simulink model "UAV_Research_Environment"  (R2025a)
settings: Solver=ode23t  StartTime=0.0  StopTime=130  MaxStep=2e-3  RelTol=1e-4  AbsTol=1e-3  EnableMultiTasking=on
InitFcn:
  | skipInitialization = false;
  | 
  | if evalin('base', ...
  |         'exist(''CONTROLLER_TUNING_ACTIVE'',''var'')')
  | 
  |     skipInitialization = evalin('base', ...
  |         'logical(CONTROLLER_TUNING_ACTIVE)');
  | end
  | 
  | if ~skipInitialization
  | 
  |     icraControllerPrepared = false;
  | 
  |     hasICRAVariables = evalin('base', ...
  |         ['exist(''AUTOPILOT'',''var'') && ' ...
  |          'exist(''ICRA_ACTIVE_CONTROLLER'',''var'') && ' ...
  |          'exist(''ICRA_ACTIVE_RUN_ID'',''var'')']);
  | 
  |     if hasICRAVariables
  | 
  |         icraControllerPrepared = evalin('base', ...
  |             ['isstruct(AUTOPILOT) && ' ...
  |              'isfield(AUTOPILOT,''info'') && ' ...
  |              'isfield(AUTOPILOT.info,''ICRAControllerID'') && ' ...
  |              'strcmp(string(AUTOPILOT.info.ICRAControllerID), ' ...
  |                     'string(ICRA_ACTIVE_CONTROLLER))']);
  | 
  |     end
  | 
  |     if icraControllerPrepared
  |         skipInitialization = true;
  |     end
  | end
  | 
  | if ~skipInitialization
  | 
  |     mdl = bdroot;
  | 
  |     mdl_file = get_param(mdl, 'FileName');
  | 
  |     project_root = fileparts(mdl_file);
  | 
  |     init_file = fullfile(project_root, 'initialize_project.m');
  | 
  |     if exist(init_file, 'file')
  | 
  |         run(init_file);
  | 
  |     else
  | 
  |         error('initialize_project.m was not found in the model folder.');
  | 
  |     end
  | end
values from neighbouring files (symbols this model uses):
  A_UAV = struct()    [UAV_analytical.m]
  AUTOPILOT = struct()    [UAV_autopilot.m]
  B_UAV = struct()    [UAV_block.m]
  D = A_UAV.source.propeller_diameter_m    [UAV_analytical.m]    (also in plot_controller_results.m = permute(                  D,                  order); plot_estimator_results.m = permute(              D,              order); plot_mission_results.m = permute(                  D,                  order); plot_touchdown_diagnostics.m = permute(                  D,                  order))
  OPERATOR_MODE = OPERATOR_MODE_MANUAL    [initialize_project.m]    (also in uav_remote_gui.m = uint8(0))
  P_ENV = struct()    [Environment.m]
  P_UAV = struct()    [UAV_simscape.m]
  s = sin(angle)    [uav_remote_gui.m]
  SENSOR = struct()    [UAV_sensors.m]
  TRAJECTORY_CONFIG = struct()    [UAV_trajectories.m]
  TRAJECTORY_ID = uint8(          trajectoryIDNumeric)    [UAV_trajectories.m]
  X = reshape(                  D,                  nt,                  [])    [plot_controller_results.m]    (also in plot_estimator_results.m = reshape(              D,              nt,              []); plot_mission_results.m; plot_touchdown_diagnostics.m; plot_trajectory_3d.m)
  Y = absolutePlanNED(1,:)    [plot_trajectory_3d.m]    (also in uav_remote_gui.m = positionNED(:,1))
  Z = landedCGDown -          absolutePlanNED(3,:)    [plot_trajectory_3d.m]    (also in uav_remote_gui.m = landedCGDown-positionNED(:,3))
undefined symbols (not defined in the file or in its folder): Acceleration_ref, F, fractalcoef, Light, MIL, Position_ref, Velocity_ref, Yaw_ref, YawRate_ref
libraries: sm_lib x49, nesl_utility x29, fl_lib x17, slpidlib x16, simulink x14, ee_lib x5, sdl_lib x4, aerolibwind2 x3, aerolibatmos2 x2, sensorbarometerlib x1, sensorgpslib x1, mspsensorlib x1
(part 9 of 9)

== matlab function UAV_Research_Environment/State Estimator/Navigation_Health ==
  data: HealthFlags input; NavValid output; StateStd input; InnovationSigma input; NavHealthStatus output; ESTIMATOR parameter
function [NavValid, NavHealthStatus] = ...
    Navigation_Health(HealthFlags, StateStd, InnovationSigma, ESTIMATOR)
persistent gpsSamplesSinceUpdate
persistent magSamplesSinceUpdate
persistent baroSamplesSinceUpdate
persistent gpsUpdateObserved
persistent magUpdateObserved
persistent baroUpdateObserved
persistent gpsInnovationHealthyLatched
persistent magInnovationHealthyLatched
persistent baroInnovationHealthyLatched
persistent healthyCounter
persistent unhealthyCounter
persistent navValidLatched
Ts = ...
    ESTIMATOR.rate.imuSampleTime_s;
gpsTimeoutSamples = ...
    uint32(ceil( ...
        ESTIMATOR.health.gpsTimeout_s / Ts));
magTimeoutSamples = ...
    uint32(ceil( ...
        ESTIMATOR.health.magTimeout_s / Ts));
baroTimeoutSamples = ...
    uint32(ceil( ...
        ESTIMATOR.health.baroTimeout_s / Ts));
validConfirmationSamples = ...
    uint32(ceil( ...
        ESTIMATOR.health.validConfirmationTime_s / Ts));
invalidConfirmationSamples = ...
    uint32(ceil( ...
        ESTIMATOR.health.invalidConfirmationTime_s / Ts));
if isempty(navValidLatched)
    gpsSamplesSinceUpdate = ...
        gpsTimeoutSamples + uint32(1);
    magSamplesSinceUpdate = ...
        magTimeoutSamples + uint32(1);
    baroSamplesSinceUpdate = ...
        baroTimeoutSamples + uint32(1);
    gpsUpdateObserved = ...
        false;
    magUpdateObserved = ...
        false;
    baroUpdateObserved = ...
        false;
    gpsInnovationHealthyLatched = ...
        false;
    magInnovationHealthyLatched = ...
        false;
    baroInnovationHealthyLatched = ...
        false;
    healthyCounter = ...
        uint32(0);
    unhealthyCounter = ...
        uint32(0);
    navValidLatched = ...
        false;
end
EstimatorInitialized = ...
    logical(HealthFlags(1));
IMUInputValid = ...
    logical(HealthFlags(2));
GPSInputValid = ...
    logical(HealthFlags(3));
MagInputValid = ...
    logical(HealthFlags(4));
BaroInputValid = ...
    logical(HealthFlags(5));
GPSUpdate = ...
    logical(HealthFlags(6));
MagUpdate = ...
    logical(HealthFlags(7));
BaroUpdate = ...
    logical(HealthFlags(8));
StateFinite = ...
    logical(HealthFlags(9));
CovarianceFinite = ...
    logical(HealthFlags(10));
QuaternionValid = ...
    logical(HealthFlags(11));
if ~EstimatorInitialized
    gpsSamplesSinceUpdate = ...
        gpsTimeoutSamples + uint32(1);
    magSamplesSinceUpdate = ...
        magTimeoutSamples + uint32(1);
    baroSamplesSinceUpdate = ...
        baroTimeoutSamples + uint32(1);
    gpsUpdateObserved = ...
        false;
    magUpdateObserved = ...
        false;
    baroUpdateObserved = ...
        false;
    gpsInnovationHealthyLatched = ...
        false;
    magInnovationHealthyLatched = ...
        false;
    baroInnovationHealthyLatched = ...
        false;
    healthyCounter = ...
        uint32(0);
    unhealthyCounter = ...
        uint32(0);
    navValidLatched = ...
        false;
    NavValid = ...
        false;
    NavHealthStatus = ...
        uint8(0);
    return;
end
if GPSUpdate && GPSInputValid
    gpsSamplesSinceUpdate = ...
        uint32(0);
    gpsUpdateObserved = ...
        true;
else
    if gpsSamplesSinceUpdate < intmax('uint32')
        gpsSamplesSinceUpdate = ...
            gpsSamplesSinceUpdate + uint32(1);
    end
end
GPSFresh = ...
    gpsUpdateObserved && ...
    gpsSamplesSinceUpdate <= gpsTimeoutSamples;
if MagUpdate && MagInputValid
    magSamplesSinceUpdate = ...
        uint32(0);
    magUpdateObserved = ...
        true;
else
    if magSamplesSinceUpdate < intmax('uint32')
        magSamplesSinceUpdate = ...
            magSamplesSinceUpdate + uint32(1);
    end
end
MagFresh = ...
    magUpdateObserved && ...
    magSamplesSinceUpdate <= magTimeoutSamples;
if BaroUpdate && BaroInputValid
    baroSamplesSinceUpdate = ...
        uint32(0);
    baroUpdateObserved = ...
        true;
else
    if baroSamplesSinceUpdate < intmax('uint32')
        baroSamplesSinceUpdate = ...
            baroSamplesSinceUpdate + uint32(1);
    end
end
BaroFresh = ...
    baroUpdateObserved && ...
    baroSamplesSinceUpdate <= baroTimeoutSamples;
if GPSUpdate && GPSInputValid
    currentGPSInnovationHealthy = ...
        true;
    for i = 1:6
        if ~isfinite(InnovationSigma(i)) || ...
                InnovationSigma(i) < 0.0 || ...
                InnovationSigma(i) > ...
                ESTIMATOR.health.gpsInnovationSigmaMax
            currentGPSInnovationHealthy = ...
                false;
        end
    end
    gpsInnovationHealthyLatched = ...
        currentGPSInnovationHealthy;
end
GPSInnovationHealthy = ...
    gpsUpdateObserved && ...
    gpsInnovationHealthyLatched;
if MagUpdate && MagInputValid
    currentMagInnovationHealthy = ...
        true;
    for i = 7:9
        if ~isfinite(InnovationSigma(i)) || ...
                InnovationSigma(i) < 0.0 || ...
                InnovationSigma(i) > ...
                ESTIMATOR.health.magInnovationSigmaMax
            currentMagInnovationHealthy = ...
                false;
        end
    end
    magInnovationHealthyLatched = ...
        currentMagInnovationHealthy;
end
MagInnovationHealthy = ...
    magUpdateObserved && ...
    magInnovationHealthyLatched;
if BaroUpdate && BaroInputValid
    currentBaroInnovationHealthy = ...
        isfinite(InnovationSigma(10)) && ...
        InnovationSigma(10) >= 0.0 && ...
        InnovationSigma(10) <= ...
        ESTIMATOR.health.baroInnovationSigmaMax;
    baroInnovationHealthyLatched = ...
        currentBaroInnovationHealthy;
end
BaroInnovationHealthy = ...
    baroUpdateObserved && ...
    baroInnovationHealthyLatched;
NumericallyHealthy = ...
    StateFinite && ...
    CovarianceFinite;
positionStdHealthy = ...
    isfinite(StateStd(1)) && ...
    isfinite(StateStd(2)) && ...
    isfinite(StateStd(3)) && ...
    StateStd(1) >= 0.0 && ...
    StateStd(2) >= 0.0 && ...
    StateStd(3) >= 0.0 && ...
    StateStd(1) <= ESTIMATOR.health.positionStdMax_m(1) && ...
    StateStd(2) <= ESTIMATOR.health.positionStdMax_m(2) && ...
    StateStd(3) <= ESTIMATOR.health.positionStdMax_m(3);
velocityStdHealthy = ...
    isfinite(StateStd(4)) && ...
    isfinite(StateStd(5)) && ...
    isfinite(StateStd(6)) && ...
    StateStd(4) >= 0.0 && ...
    StateStd(5) >= 0.0 && ...
    StateStd(6) >= 0.0 && ...
    StateStd(4) <= ESTIMATOR.health.velocityStdMax_m_s(1) && ...
    StateStd(5) <= ESTIMATOR.health.velocityStdMax_m_s(2) && ...
    StateStd(6) <= ESTIMATOR.health.velocityStdMax_m_s(3);
StateUncertaintyHealthy = ...
    positionStdHealthy && ...
    velocityStdHealthy;
allHealthy = ...
    NumericallyHealthy && ...
    IMUInputValid && ...
    QuaternionValid && ...
    GPSFresh && ...
    MagFresh && ...
    BaroFresh && ...
    StateUncertaintyHealthy && ...
    GPSInnovationHealthy && ...
    MagInnovationHealthy && ...
    BaroInnovationHealthy;
if ~NumericallyHealthy
    NavHealthStatus = ...
        uint8(5);
elseif ~QuaternionValid
    NavHealthStatus = ...
        uint8(9);
elseif ~IMUInputValid
    NavHealthStatus = ...
        uint8(2);
elseif ~GPSFresh
    NavHealthStatus = ...
        uint8(3);
elseif ~MagFresh
    NavHealthStatus = ...
        uint8(4);
elseif ~BaroFresh
    NavHealthStatus = ...
        uint8(10);
elseif ~StateUncertaintyHealthy
    NavHealthStatus = ...
        uint8(6);
elseif ~GPSInnovationHealthy
    NavHealthStatus = ...
        uint8(7);
elseif ~MagInnovationHealthy
    NavHealthStatus = ...
        uint8(8);
elseif ~BaroInnovationHealthy
    NavHealthStatus = ...
        uint8(11);
else
    NavHealthStatus = ...
        uint8(1);
end
criticalFailure = ...
    ~NumericallyHealthy || ...
    ~IMUInputValid || ...
    ~QuaternionValid;
if criticalFailure
    navValidLatched = ...
        false;
    healthyCounter = ...
        uint32(0);
    unhealthyCounter = ...
        uint32(0);
elseif allHealthy
    unhealthyCounter = ...
        uint32(0);
    if healthyCounter < validConfirmationSamples
        healthyCounter = ...
            healthyCounter + uint32(1);
    end
    if healthyCounter >= validConfirmationSamples
        navValidLatched = ...
            true;
    end
else
    healthyCounter = ...
        uint32(0);
    if unhealthyCounter < invalidConfirmationSamples
        unhealthyCounter = ...
            unhealthyCounter + uint32(1);
    end
    if unhealthyCounter >= invalidConfirmationSamples
        navValidLatched = ...
            false;
    end
end
NavValid = ...
    navValidLatched;
end

== matlab function UAV_Research_Environment/Autopilot/Flight Control/Reference Supervisor/Failsafe_Reference ==
  data: Position_ref input; Position_ref_eff output; Velocity_ref input; Acceleration_ref input; Yaw_ref input; YawRate_ref input; Position_est input; Euler_est input; mode input; navFailsafe input; descentRate input; Velocity_ref_eff output; Acceleration_ref_eff output; Yaw_ref_eff output; YawRate_ref_eff output
function [Position_ref_eff, Velocity_ref_eff, Acceleration_ref_eff, ...
          Yaw_ref_eff, YawRate_ref_eff] = ...
    Failsafe_Reference(Position_ref, Velocity_ref, Acceleration_ref, ...
                       Yaw_ref, YawRate_ref, Position_est, Euler_est, ...
                       mode, navFailsafe, descentRate)

Position_ref_eff = Position_ref;
Velocity_ref_eff = Velocity_ref;
Acceleration_ref_eff = Acceleration_ref;
Yaw_ref_eff = Yaw_ref;
YawRate_ref_eff = YawRate_ref;

if mode == navFailsafe

    Position_ref_eff = Position_est;
    Velocity_ref_eff = [0; 0; descentRate];
    Acceleration_ref_eff = [0; 0; 0];
    Yaw_ref_eff = Euler_est(3);
    YawRate_ref_eff = 0;

end

end

== matlab function UAV_Research_Environment/Control Ground Station/Mission Plan/Generate_Mission_Plan ==
  data: HomePosition input; MissionPlan output; NumWaypoints output; MissionHome output; MissionPlanRelative input; NumWaypointsIn input
function [MissionPlan, NumWaypoints, MissionHome] = ...
    Generate_Mission_Plan( ...
        HomePosition, ...
        MissionPlanRelative, ...
        NumWaypointsIn)

maxWaypoints = ...
    size( ...
        MissionPlanRelative, ...
        2);

MissionPlan = ...
    zeros( ...
        4, ...
        maxWaypoints);

NumWaypoints = ...
    uint16(0);

homeValid = ...
    numel(HomePosition) == 3 && ...
    isfinite(HomePosition(1)) && ...
    isfinite(HomePosition(2)) && ...
    isfinite(HomePosition(3));

if homeValid

    H = ...
        [ ...
            double(HomePosition(1));
            double(HomePosition(2));
            double(HomePosition(3))
        ];

else

    H = ...
        zeros(3,1);

end

MissionHome = ...
    H;

bufferValid = ...
    size(MissionPlanRelative,1) == 4 && ...
    maxWaypoints >= 1;

if ~bufferValid

    return;

end

numWaypointsRaw = ...
    double( ...
        NumWaypointsIn);

numWaypointsValid = ...
    isscalar(numWaypointsRaw) && ...
    isfinite(numWaypointsRaw) && ...
    numWaypointsRaw >= 1 && ...
    numWaypointsRaw <= maxWaypoints && ...
    abs( ...
        numWaypointsRaw - ...
        round(numWaypointsRaw)) < 1e-12;

if ~numWaypointsValid

    return;

end

numWaypointsDouble = ...
    round( ...
        numWaypointsRaw);

NumWaypoints = ...
    uint16( ...
        numWaypointsDouble);

activePlanValid = ...
    true;

for waypointIndex = 1:maxWaypoints

    if waypointIndex <= numWaypointsDouble

        for rowIndex = 1:4

            if ~isfinite( ...
                    MissionPlanRelative( ...
                        rowIndex, ...
                        waypointIndex))

                activePlanValid = ...
                    false;

            end

        end

    end

end

if ~activePlanValid

    MissionPlan(:) = ...
        0.0;

    NumWaypoints = ...
        uint16(0);

    return;

end

for waypointIndex = 1:maxWaypoints

    if waypointIndex <= numWaypointsDouble

        MissionPlan(1,waypointIndex) = ...
            H(1) + ...
            double( ...
                MissionPlanRelative( ...
                    1, ...
                    waypointIndex));

        MissionPlan(2,waypointIndex) = ...
            H(2) + ...
            double( ...
                MissionPlanRelative( ...
                    2, ...
                    waypointIndex));

        MissionPlan(3,waypointIndex) = ...
            H(3) + ...
            double( ...
                MissionPlanRelative( ...
                    3, ...
                    waypointIndex));

        yawReference = ...
            double( ...
                MissionPlanRelative( ...
                    4, ...
                    waypointIndex));

        MissionPlan(4,waypointIndex) = ...
            atan2( ...
                sin(yawReference), ...
                cos(yawReference));

    end

end

end

== matlab function UAV_Research_Environment/UAV Plant/UAV Block [Simulink Blocks]/Ground_Contact_Model ==
  data: p_ned input; F_ground_body output; v_ned input; R_BN input; Omega_body input; Tau_ground_body output; UAV_CONTACT parameter
function [F_ground_body, Tau_ground_body] = ...
    Ground_Contact_Model( ...
        p_ned, ...
        v_ned, ...
        R_BN, ...
        Omega_body, ...
        UAV_CONTACT)
F_ground_body = ...
    zeros(3,1);
Tau_ground_body = ...
    zeros(3,1);
kGround = ...
    UAV_CONTACT.stiffness_N_m;
cGround = ...
    UAV_CONTACT.damping_N_s_m;
muStatic = ...
    UAV_CONTACT.static_friction;
muDynamic = ...
    UAV_CONTACT.dynamic_friction;
vCritical = ...
    UAV_CONTACT.critical_velocity_m_s;
if vCritical < 1e-6
    vCritical = ...
        1e-6;
end
groundDown = ...
    UAV_CONTACT.ground_down_m;
for i = 1:4
    r_body = [ ...
        UAV_CONTACT.arm_body_m(i,1);
        UAV_CONTACT.arm_body_m(i,2);
        UAV_CONTACT.arm_body_m(i,3)];
    r_ned = ...
        R_BN * r_body;
    p_contact_ned = ...
        p_ned + r_ned;
    v_rot_body = ...
        cross( ...
            Omega_body, ...
            r_body);
    v_rot_ned = ...
        R_BN * v_rot_body;
    v_contact_ned = ...
        v_ned + ...
        v_rot_ned;
    penetration = ...
        p_contact_ned(3) - ...
        groundDown;
    if penetration > 0.0
        penetrationRate = ...
            v_contact_ned(3);
        normalForce = ...
            kGround * penetration + ...
            cGround * penetrationRate;
        if normalForce < 0.0
            normalForce = ...
                0.0;
        end
        vNorth = ...
            v_contact_ned(1);
        vEast = ...
            v_contact_ned(2);
        tangentialSpeed = ...
            sqrt( ...
                vNorth*vNorth + ...
                vEast*vEast);
        velocityRatio = ...
            tangentialSpeed / ...
            vCritical;
        mu = ...
            muDynamic + ...
            (muStatic - muDynamic) * ...
            exp( ...
                -(velocityRatio * velocityRatio));
        denominator = ...
            sqrt( ...
                tangentialSpeed*tangentialSpeed + ...
                vCritical*vCritical);
        frictionNorth = ...
           -mu * normalForce * ...
            vNorth / ...
            denominator;
        frictionEast = ...
           -mu * normalForce * ...
            vEast / ...
            denominator;
        F_contact_ned = [ ...
            frictionNorth;
            frictionEast;
           -normalForce];
        F_contact_body = ...
            R_BN.' * ...
            F_contact_ned;
        F_ground_body = ...
            F_ground_body + ...
            F_contact_body;
        Tau_contact_body = ...
            cross( ...
                r_body, ...
                F_contact_body);
        Tau_ground_body = ...
            Tau_ground_body + ...
            Tau_contact_body;
    end
end
end

== matlab function UAV_Research_Environment/UAV Plant/UAV Physical [Simscape]/yaw adapter ==
  data: Omega input; P1 output; P2 output; P3 output; P4 output
function [P1, P2, P3, P4] = fcn(Omega)

omega = reshape(Omega, 4, 1);

yawVector = ...
    [-1.0; ...
     -1.0; ...
      1.0; ...
      1.0];

yawComponent = ...
    0.25 * ...
    (yawVector.' * omega);

omegaL3 = ...
    omega - ...
    2.0 * yawComponent * yawVector;

P1 = omegaL3(1);

P2 = omegaL3(2);

P3 = omegaL3(3);

P4 = omegaL3(4);

end

== matlab function UAV_Research_Environment/Plots & Metrics/Estimator Comparison/Euler_Error ==
  data: Euler_true input; EulerError output; Euler_est input
function EulerError = Euler_Error(Euler_true,Euler_est)
%#codegen

d = Euler_est - Euler_true;
EulerError = atan2(sin(d),cos(d));

end

== matlab function UAV_Research_Environment/State Estimator/INS_EKF ==
  data: Accel input size=[3 1]; Position output size=[3 1]; Gyro input size=[3 1]; LLA input size=[3 1]; MagneticField input size=[3 1]; GPSVelocity input size=[3 1]; BaroAltitude input; Velocity output size=[3 1]; Q output size=[4 1]; AngularRate output; Acceleration output; ESTIMATOR parameter; GyroBias output; AccelBias output; MagBias output; HealthFlags output; StateStd output; InnovationSigma output
function [Position, Velocity, Q, AngularRate, Acceleration, ...
    GyroBias, AccelBias, MagBias, ...
    HealthFlags, StateStd, InnovationSigma] = ...
    INS_EKF(Accel, Gyro, LLA, MagneticField, GPSVelocity, ...
            BaroAltitude, ESTIMATOR)
persistent F
persistent filterInitialized
persistent imuCounter
persistent gpsInitPositionBuffer
persistent gpsInitVelocityBuffer
persistent gpsInitCount
persistent baroInitBuffer
persistent baroInitCount
persistent gpsInnovationSigmaLast
persistent magInnovationSigmaLast
persistent baroInnovationSigmaLast
IMU_RATE_HZ = ...
    ESTIMATOR.rate.imu_Hz;
Ts = ...
    ESTIMATOR.rate.imuSampleTime_s;
GPS_DIV = uint32( ...
    ESTIMATOR.rate.gpsDivisor);
MAG_DIV = uint32( ...
    ESTIMATOR.rate.magDivisor);
BARO_DIV = uint32( ...
    ESTIMATOR.rate.baroDivisor);
REFERENCE_LLA = reshape( ...
    ESTIMATOR.reference.lla_deg_m, ...
    1, ...
    3);
GRAVITY_NED = reshape( ...
    ESTIMATOR.gravity.ned_m_s2, ...
    3, ...
    1);
ROBUST_POSITION_P0_SCALE_NE = ...
    double( ...
        ESTIMATOR.initial.robustCovarianceScale.position_NE);
ROBUST_POSITION_P0_SCALE_D = ...
    double( ...
        ESTIMATOR.initial.robustCovarianceScale.position_D);
ROBUST_VELOCITY_P0_SCALE_NE = ...
    double( ...
        ESTIMATOR.initial.robustCovarianceScale.velocity_NE);
ROBUST_VELOCITY_P0_SCALE_D = ...
    double( ...
        ESTIMATOR.initial.robustCovarianceScale.velocity_D);
if ~isscalar(ROBUST_POSITION_P0_SCALE_NE) || ...
        ~isfinite(ROBUST_POSITION_P0_SCALE_NE) || ...
        ROBUST_POSITION_P0_SCALE_NE <= 0.0
    error( ...
        'QuadrotorFramework:InvalidRobustPositionP0ScaleNE', ...
        ['ESTIMATOR.initial.robustCovarianceScale.position_NE ', ...
         'must be a finite positive scalar.']);
end
if ~isscalar(ROBUST_POSITION_P0_SCALE_D) || ...
        ~isfinite(ROBUST_POSITION_P0_SCALE_D) || ...
        ROBUST_POSITION_P0_SCALE_D <= 0.0
    error( ...
        'QuadrotorFramework:InvalidRobustPositionP0ScaleD', ...
        ['ESTIMATOR.initial.robustCovarianceScale.position_D ', ...
         'must be a finite positive scalar.']);
end
if ~isscalar(ROBUST_VELOCITY_P0_SCALE_NE) || ...
        ~isfinite(ROBUST_VELOCITY_P0_SCALE_NE) || ...
        ROBUST_VELOCITY_P0_SCALE_NE <= 0.0
    error( ...
        'QuadrotorFramework:InvalidRobustVelocityP0ScaleNE', ...
        ['ESTIMATOR.initial.robustCovarianceScale.velocity_NE ', ...
         'must be a finite positive scalar.']);
end
if ~isscalar(ROBUST_VELOCITY_P0_SCALE_D) || ...
        ~isfinite(ROBUST_VELOCITY_P0_SCALE_D) || ...
        ROBUST_VELOCITY_P0_SCALE_D <= 0.0
    error( ...
        'QuadrotorFramework:InvalidRobustVelocityP0ScaleD', ...
        ['ESTIMATOR.initial.robustCovarianceScale.velocity_D ', ...
         'must be a finite positive scalar.']);
end
gpsInitSamplesConfigured = ...
    double( ...
        ESTIMATOR.initialization.gpsSamples);
baroInitSamplesConfigured = ...
    double( ...
        ESTIMATOR.initialization.baroSamples);
if ~isscalar(gpsInitSamplesConfigured) || ...
        ~isfinite(gpsInitSamplesConfigured) || ...
        gpsInitSamplesConfigured < 1 || ...
        gpsInitSamplesConfigured ~= floor(gpsInitSamplesConfigured)
    error( ...
        'QuadrotorFramework:InvalidGPSInitializationSamples', ...
        ['ESTIMATOR.initialization.gpsSamples must be a ', ...
         'positive integer.']);
end
if ~isscalar(baroInitSamplesConfigured) || ...
        ~isfinite(baroInitSamplesConfigured) || ...
        baroInitSamplesConfigured < 1 || ...
        baroInitSamplesConfigured ~= floor(baroInitSamplesConfigured)
    error( ...
        'QuadrotorFramework:InvalidBarometerInitializationSamples', ...
        ['ESTIMATOR.initialization.baroSamples must be a ', ...
         'positive integer.']);
end
GPS_INIT_SAMPLES = ...
    uint32( ...
        gpsInitSamplesConfigured);
BARO_INIT_SAMPLES = ...
    uint32( ...
        baroInitSamplesConfigured);
GPS_INIT_SAMPLES_DOUBLE = ...
    double(GPS_INIT_SAMPLES);
BARO_INIT_SAMPLES_DOUBLE = ...
    double(BARO_INIT_SAMPLES);
RposOriginal = ...
    ESTIMATOR.measurement.Rpos_m2;
Rvel = ...
    ESTIMATOR.measurement.Rvel_m2_s2;
Rmag = ...
    ESTIMATOR.measurement.Rmag_uT2;
Rbaro = ...
    ESTIMATOR.measurement.Rbaro_m2;
RposGPS = ...
    RposOriginal;
RposGPS(3,3) = ...
    1.0e6;
accel = reshape( ...
    Accel, ...
    1, ...
    3);
gyro = reshape( ...
    Gyro, ...
    1, ...
    3);
mag = reshape( ...
    MagneticField, ...
    1, ...
    3);
gpsLLA = reshape( ...
    LLA, ...
    1, ...
    3);
gpsVel = reshape( ...
    GPSVelocity, ...
    1, ...
    3);
baroAltitude = ...
    BaroAltitude(1);
IMUInputValid = ...
    isfinite(accel(1)) && ...
    isfinite(accel(2)) && ...
    isfinite(accel(3)) && ...
    isfinite(gyro(1))  && ...
    isfinite(gyro(2))  && ...
    isfinite(gyro(3));
gpsFinite = ...
    isfinite(gpsLLA(1)) && ...
    isfinite(gpsLLA(2)) && ...
    isfinite(gpsLLA(3)) && ...
    isfinite(gpsVel(1)) && ...
    isfinite(gpsVel(2)) && ...
    isfinite(gpsVel(3));
gpsLatitudeValid = ...
    gpsLLA(1) >= -90.0 && ...
    gpsLLA(1) <= 90.0;
gpsLongitudeValid = ...
    gpsLLA(2) >= -180.0 && ...
    gpsLLA(2) <= 180.0;
GPSInputValid = ...
    gpsFinite && ...
    gpsLatitudeValid && ...
    gpsLongitudeValid;
MagInputValid = ...
    isfinite(mag(1)) && ...
    isfinite(mag(2)) && ...
    isfinite(mag(3));
BaroInputValid = ...
    isfinite(baroAltitude);
if BaroInputValid
    baroDown = ...
        -(baroAltitude - REFERENCE_LLA(3));
else
    baroDown = ...
        0.0;
end
if isempty(F)
    F = insfilterMARG( ...
        'ReferenceFrame', ...
        'NED');
    F.IMUSampleRate = ...
        IMU_RATE_HZ;
    F.ReferenceLocation = ...
        REFERENCE_LLA;
    F.GyroscopeNoise = reshape( ...
        ESTIMATOR.process.GyroscopeNoise, ...
        1, ...
        3);
    F.GyroscopeBiasNoise = reshape( ...
        ESTIMATOR.process.GyroscopeBiasNoise, ...
        1, ...
        3);
    F.AccelerometerNoise = reshape( ...
        ESTIMATOR.process.AccelerometerNoise, ...
        1, ...
        3);
    F.AccelerometerBiasNoise = reshape( ...
        ESTIMATOR.process.AccelerometerBiasNoise, ...
        1, ...
        3);
    F.MagnetometerBiasNoise = reshape( ...
        ESTIMATOR.process.MagnetometerBiasNoise, ...
        1, ...
        3);
    F.GeomagneticVectorNoise = reshape( ...
        ESTIMATOR.process.GeomagneticVectorNoise, ...
        1, ...
        3);
    F.State = ...
        ESTIMATOR.initial.state;
    F.StateCovariance = ...
        ESTIMATOR.initial.StateCovariance;
end
if isempty(filterInitialized)
    filterInitialized = ...
        false;
end
if isempty(imuCounter)
    imuCounter = ...
        uint32(0);
end
if isempty(gpsInitPositionBuffer)
    gpsInitPositionBuffer = ...
        zeros( ...
            GPS_INIT_SAMPLES_DOUBLE, ...
            3);
end
if isempty(gpsInitVelocityBuffer)
    gpsInitVelocityBuffer = ...
        zeros( ...
            GPS_INIT_SAMPLES_DOUBLE, ...
            3);
end
if isempty(gpsInitCount)
    gpsInitCount = ...
        uint32(0);
end
if isempty(baroInitBuffer)
    baroInitBuffer = ...
        zeros( ...
            BARO_INIT_SAMPLES_DOUBLE, ...
            1);
end
if isempty(baroInitCount)
    baroInitCount = ...
        uint32(0);
end
if isempty(gpsInnovationSigmaLast)
    gpsInnovationSigmaLast = ...
        inf(6,1);
end
if isempty(magInnovationSigmaLast)
    magInnovationSigmaLast = ...
        inf(3,1);
end
if isempty(baroInnovationSigmaLast)
    baroInnovationSigmaLast = ...
        inf;
end
GPSUpdateDue = ...
    mod( ...
        imuCounter, ...
        GPS_DIV) == 0;
MagUpdateDue = ...
    mod( ...
        imuCounter, ...
        MAG_DIV) == 0;
BaroUpdateDue = ...
    mod( ...
        imuCounter, ...
        BARO_DIV) == 0;
justInitialized = ...
    false;
if ~filterInitialized
    if GPSUpdateDue && ...
            GPSInputValid && ...
            gpsInitCount < GPS_INIT_SAMPLES
        gpsPositionNED = ...
            lla2ned( ...
                gpsLLA, ...
                REFERENCE_LLA, ...
                'flat');
        bufferIndex = ...
            double(gpsInitCount) + 1;
        gpsInitPositionBuffer(bufferIndex,:) = ...
            gpsPositionNED;
        gpsInitVelocityBuffer(bufferIndex,:) = ...
            gpsVel;
        gpsInitCount = ...
            gpsInitCount + ...
            uint32(1);
    end
    if BaroUpdateDue && ...
            BaroInputValid && ...
            baroInitCount < BARO_INIT_SAMPLES
        bufferIndex = ...
            double(baroInitCount) + 1;
        baroInitBuffer(bufferIndex) = ...
            baroDown;
        baroInitCount = ...
            baroInitCount + ...
            uint32(1);
    end
    if gpsInitCount >= GPS_INIT_SAMPLES && ...
            baroInitCount >= BARO_INIT_SAMPLES
        x0 = ...
            ESTIMATOR.initial.state;
        x0(1:4) = ...
            ESTIMATOR.initial.state(1:4);
        initialGPSPositionNED = ...
            median( ...
                gpsInitPositionBuffer( ...
                    1:GPS_INIT_SAMPLES_DOUBLE, ...
                    :), ...
                1);
        x0(5) = ...
            initialGPSPositionNED(1);
        x0(6) = ...
            initialGPSPositionNED(2);
        initialBaroDown = ...
            median( ...
                baroInitBuffer( ...
                    1:BARO_INIT_SAMPLES_DOUBLE));
        x0(7) = ...
            initialBaroDown;
        initialVelocityNED = ...
            median( ...
                gpsInitVelocityBuffer( ...
                    1:GPS_INIT_SAMPLES_DOUBLE, ...
                    :), ...
                1);
        x0(8:10) = ...
            initialVelocityNED(:);
        x0(11:13) = ...
            ESTIMATOR.initial.state(11:13);
        x0(14:16) = ...
            ESTIMATOR.initial.state(14:16);
        x0(17:19) = ...
            ESTIMATOR.initial.state(17:19);
        x0(20:22) = ...
            ESTIMATOR.initial.state(20:22);
        P0 = ...
            ESTIMATOR.initial.StateCovariance;
        gpsMedianVarianceFactor = ...
            1.5707963267948966 / ...
            GPS_INIT_SAMPLES_DOUBLE;
        baroMedianVarianceFactor = ...
            1.5707963267948966 / ...
            BARO_INIT_SAMPLES_DOUBLE;
        P0(5,5) = ...
            ROBUST_POSITION_P0_SCALE_NE * ...
            RposOriginal(1,1) * ...
            gpsMedianVarianceFactor;
        P0(6,6) = ...
            ROBUST_POSITION_P0_SCALE_NE * ...
            RposOriginal(2,2) * ...
            gpsMedianVarianceFactor;
        P0(7,7) = ...
            ROBUST_POSITION_P0_SCALE_D * ...
            Rbaro * ...
            baroMedianVarianceFactor;
        P0(8,8) = ...
            ROBUST_VELOCITY_P0_SCALE_NE * ...
            Rvel(1,1) * ...
            gpsMedianVarianceFactor;
        P0(9,9) = ...
            ROBUST_VELOCITY_P0_SCALE_NE * ...
            Rvel(2,2) * ...
            gpsMedianVarianceFactor;
        P0(10,10) = ...
            ROBUST_VELOCITY_P0_SCALE_D * ...
            Rvel(3,3) * ...
            gpsMedianVarianceFactor;
        robustCovarianceValid = ...
            isfinite(P0(5,5))  && P0(5,5)  >= 0.0 && ...
            isfinite(P0(6,6))  && P0(6,6)  >= 0.0 && ...
            isfinite(P0(7,7))  && P0(7,7)  >= 0.0 && ...
            isfinite(P0(8,8))  && P0(8,8)  >= 0.0 && ...
            isfinite(P0(9,9))  && P0(9,9)  >= 0.0 && ...
            isfinite(P0(10,10)) && P0(10,10) >= 0.0;
        if ~robustCovarianceValid
            error( ...
                'QuadrotorFramework:InvalidRobustInitialCovariance', ...
                ['Robust estimator initialization generated an ', ...
                 'invalid position/velocity covariance.']);
        end
        F.State = ...
            x0;
        F.StateCovariance = ...
            P0;
        filterInitialized = ...
            true;
        justInitialized = ...
            true;
    end
end
EstimatorInitialized = ...
    filterInitialized;
GPSUpdate = ...
    false;
MagUpdate = ...
    false;
BaroUpdate = ...
    false;
if EstimatorInitialized
    if ~justInitialized && ...
            IMUInputValid
        predict( ...
            F, ...
            accel, ...
            gyro);
    end
    if ~justInitialized && ...
            MagUpdateDue && ...
            MagInputValid
        [magResidual, magResidualCovariance] = ...
            fusemag( ...
                F, ...
                mag, ...
                Rmag);
        MagUpdate = ...
            true;
        for i = 1:3
            innovationVariance = ...
                magResidualCovariance(i,i);
            if isfinite(innovationVariance) && ...
                    innovationVariance > 1e-12
                magInnovationSigmaLast(i) = ...
                    abs(magResidual(i)) / ...
                    sqrt(innovationVariance);
            else
                magInnovationSigmaLast(i) = ...
                    inf;
            end
        end
    end
    if ~justInitialized && ...
            GPSUpdateDue && ...
            GPSInputValid
        [gpsResidual, gpsResidualCovariance] = ...
            fusegps( ...
                F, ...
                gpsLLA, ...
                RposGPS, ...
                gpsVel, ...
                Rvel);
        GPSUpdate = ...
            true;
        for i = 1:6
            innovationVariance = ...
                gpsResidualCovariance(i,i);
            if isfinite(innovationVariance) && ...
                    innovationVariance > 1e-12
                gpsInnovationSigmaLast(i) = ...
                    abs(gpsResidual(i)) / ...
                    sqrt(innovationVariance);
            else
                gpsInnovationSigmaLast(i) = ...
                    inf;
            end
        end
    end
    if ~justInitialized && ...
            BaroUpdateDue && ...
            BaroInputValid
        [baroResidual, baroResidualCovariance] = ...
            residual( ...
                F, ...
                7, ...
                baroDown, ...
                Rbaro);
        correct( ...
            F, ...
            7, ...
            baroDown, ...
            Rbaro);
        BaroUpdate = ...
            true;
        innovationVariance = ...
            baroResidualCovariance(1,1);
        if isfinite(innovationVariance) && ...
                innovationVariance > 1e-12
            baroInnovationSigmaLast = ...
                abs(baroResidual(1)) / ...
                sqrt(innovationVariance);
        else
            baroInnovationSigmaLast = ...
                inf;
        end
    end
end
imuCounter = ...
    imuCounter + ...
    uint32(1);
if EstimatorInitialized
    x = ...
        F.State;
    P = ...
        F.StateCovariance;
else
    x = ...
        ESTIMATOR.initial.state;
    P = ...
        ESTIMATOR.initial.StateCovariance;
end
StateFinite = ...
    true;
for i = 1:22
    if ~isfinite(x(i))
        StateFinite = ...
            false;
    end
end
CovarianceFinite = ...
    true;
for row = 1:22
    for column = 1:22
        if ~isfinite(P(row,column))
            CovarianceFinite = ...
                false;
        end
    end
end
Position = ...
    x(5:7);
Velocity = ...
    x(8:10);
PositionStd = ...
    zeros(3,1);
for i = 1:3
    variance = ...
        P(i + 4, ...
          i + 4);
    if isfinite(variance) && ...
            variance >= 0.0
        PositionStd(i) = ...
            sqrt(variance);
    else
        PositionStd(i) = ...
            inf;
    end
end
VelocityStd = ...
    zeros(3,1);
for i = 1:3
    variance = ...
        P(i + 7, ...
          i + 7);
    if isfinite(variance) && ...
            variance >= 0.0
        VelocityStd(i) = ...
            sqrt(variance);
    else
        VelocityStd(i) = ...
            inf;
    end
end
Q_filter = ...
    x(1:4);
qNorm = sqrt( ...
    Q_filter(1)*Q_filter(1) + ...
    Q_filter(2)*Q_filter(2) + ...
    Q_filter(3)*Q_filter(3) + ...
    Q_filter(4)*Q_filter(4));
QuaternionValid = ...
    isfinite(qNorm) && ...
    qNorm > 1e-12;
if QuaternionValid
    Q_filter = ...
        Q_filter / ...
        qNorm;
end
Q = ...
    Q_filter;
deltaAngleBias = ...
    x(11:13);
GyroBias = ...
    deltaAngleBias / ...
    Ts;
gyroBody = reshape( ...
    Gyro, ...
    3, ...
    1);
AngularRate = ...
    gyroBody - ...
    GyroBias;
deltaVelocityBias = ...
    x(14:16);
AccelBias = ...
    deltaVelocityBias / ...
    Ts;
MagBias = ...
    x(20:22);
accelBody = reshape( ...
    Accel, ...
    3, ...
    1);
accelBodyCorrected = ...
    accelBody - ...
    AccelBias;
qw = ...
    Q_filter(1);
qx = ...
    Q_filter(2);
qy = ...
    Q_filter(3);
qz = ...
    Q_filter(4);
C_nb = [ ...
    1 - 2*(qy*qy + qz*qz), ...
        2*(qx*qy - qw*qz), ...
        2*(qx*qz + qw*qy); ...
    ...
        2*(qx*qy + qw*qz), ...
    1 - 2*(qx*qx + qz*qz), ...
        2*(qy*qz - qw*qx); ...
    ...
        2*(qx*qz - qw*qy), ...
        2*(qy*qz + qw*qx), ...
    1 - 2*(qx*qx + qy*qy)];
if ESTIMATOR.acceleration.gravityCompensation
    Acceleration = ...
        GRAVITY_NED - ...
        C_nb * accelBodyCorrected;
else
    Acceleration = ...
        -C_nb * accelBodyCorrected;
end
HealthFlags = ...
    false(11,1);
HealthFlags(1) = ...
    EstimatorInitialized;
HealthFlags(2) = ...
    IMUInputValid;
HealthFlags(3) = ...
    GPSInputValid;
HealthFlags(4) = ...
    MagInputValid;
HealthFlags(5) = ...
    BaroInputValid;
HealthFlags(6) = ...
    GPSUpdate;
HealthFlags(7) = ...
    MagUpdate;
HealthFlags(8) = ...
    BaroUpdate;
HealthFlags(9) = ...
    StateFinite;
HealthFlags(10) = ...
    CovarianceFinite;
HealthFlags(11) = ...
    QuaternionValid;
StateStd = [ ...
    PositionStd(1);
    PositionStd(2);
    PositionStd(3);
    VelocityStd(1);
    VelocityStd(2);
    VelocityStd(3)];
InnovationSigma = [ ...
    gpsInnovationSigmaLast(1);
    gpsInnovationSigmaLast(2);
    gpsInnovationSigmaLast(3);
    gpsInnovationSigmaLast(4);
    gpsInnovationSigmaLast(5);
    gpsInnovationSigmaLast(6);
    magInnovationSigmaLast(1);
    magInnovationSigmaLast(2);
    magInnovationSigmaLast(3);
    baroInnovationSigmaLast];
end

== matlab function UAV_Research_Environment/Plots & Metrics/Estimator Comparison/Quaternion_Attitude_Error ==
  data: Q_true input; AttitudeErrorNorm output; Q_est input
function AttitudeErrorNorm = Quaternion_Attitude_Error(Q_true,Q_est)
%#codegen

qt = reshape(Q_true,4,1);
qe = reshape(Q_est,4,1);

qt = qt / max(norm(qt),eps);
qe = qe / max(norm(qe),eps);

c = abs(dot(qt,qe));
c = min(max(c,0),1);

AttitudeErrorNorm = 2 * acos(c);

end
